simulink model "em_blocks"  (R2025a)
settings: Solver=VariableStepAuto  StartTime=0.0  StopTime=10.0  RelTol=1e-3
libraries: simulink x1
settings Model: Creator=ROHAN A S GOWDA  LastModifiedBy=ROHAN A S GOWDA

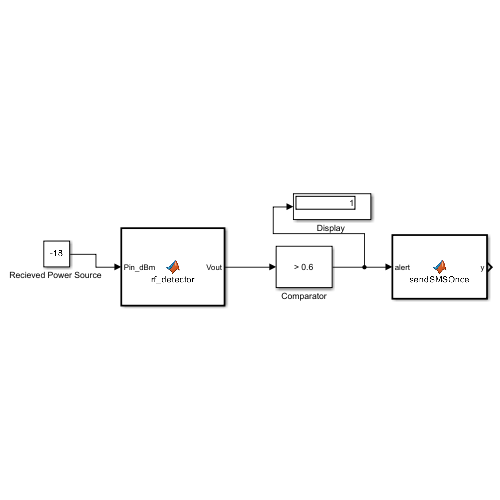
[thumbnail: Simulink's stored preview of the top-level diagram]
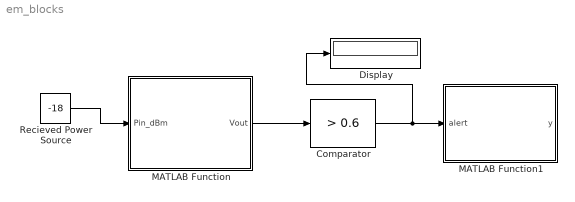
== system em_blocks ==
  Comparator : simulink/Logic and Bit Operations/Compare To Constant  relop=>  const=0.6  OutDataTypeStr=boolean
  "Display " : Display
  MATLAB Function : MATLAB Function  TreatAsAtomicUnit=on
  MATLAB Function1 : MATLAB Function  TreatAsAtomicUnit=on
  "Recieved Power Source " : Constant  Value=-18  OutDataTypeStr=double
  wires:
  MATLAB Function/1(Vout) -> Comparator/1
  Comparator/1 -> "Display "/1, MATLAB Function1/1(alert)
  "Recieved Power Source "/1 -> MATLAB Function/1(Pin_dBm)

== matlab function em_blocks/MATLAB Function ==
  data: Pin_dBm input; Vout output
function Vout = rf_detector(Pin_dBm)
    slope     = 0.025;
    intercept = 0.85;
    Vout      = intercept + slope * (Pin_dBm + 10);
end

== matlab function em_blocks/MATLAB Function1 ==
  data: alert input; y output
function y = sendSMSOnce(alert)
%#codegen
coder.extrinsic('sendTwilioSMS');  % ✅ MUST be at the top level
persistent alreadySent
if isempty(alreadySent)
    alreadySent = false;
end

y = 0; % Default output

if alert && ~alreadySent
    sendTwilioSMS();      % Call external function
    alreadySent = true;   % Prevent future triggers
    y = 1;
end
